simulink model "HallSensorTest"  (R2023b)
settings: Solver=FixedStepAuto  StartTime=0.0  StopTime=inf  FixedStep=0.01  RelTol=1e-3  EnableMultiTasking=on
libraries: aerolibconvert2 x1, simulink x1
settings Model: SimulationMode=external  ExtModeTrigDuration=2  Creator=sword  LastModifiedBy=sword
settings SolverCC: AutoInsertRateTranBlk=on
settings DataIOCC: SaveFormat=StructureWithTime  DSMLogging=off
settings OptimizationCC: DefaultUnderspecifiedDataType=single  EnhancedBackFolding=on  PassReuseOutputArgsAs=Individual arguments  ZeroExternalMemoryAtStartup=off  ZeroInternalMemoryAtStartup=off  MaxStackSize=64  OptimizeBlockOrder=speed  DifferentSizesBufferReuse=on  OptimizationCustomize=off  EfficientTunableParamExpr=on
settings DebuggingCC: MultiTaskDSMMsg=none  ParameterPrecisionLossMsg=none  ParameterTunabilityLossMsg=error
settings HardwareCC: ProdBitPerInt=16  ProdBitPerPointer=16  ProdBitPerSizeT=16  ProdBitPerPtrDiffT=16  ProdLargestAtomicFloat=None  ProdWordSize=8  ProdHWDeviceType=Atmel->AVR
settings SFSimCC: MATLABDynamicMemAlloc=off
settings RTWCC: Description=Embedded Coder  SystemTargetFile=ert.tlc  HardwareBoard=Arduino Mega ADK  TemplateMakefile=ert_default_tmf  Toolchain=Arduino AVR  BuildConfiguration=Faster Runs
settings CodeAppCC: ForceParamTrailComments=on  IgnoreCustomStorageClasses=off  OperatorAnnotations=on  SimulinkDataObjDesc=on  SFDataObjDesc=on  InsertBlockDesc=on
settings ERTTargetCC: SupportContinuousTime=on  SupportNonInlinedSFcns=on  SupportVariableSizeSignals=on  ExtMode=on  ExtModeTransport=3  ExtModeStaticAlloc=on  ExtModeAutomaticAllocSize=off  ExtModeStaticAllocSize=2048  ExtModeMexFile=ext_xcp  ExtModeMexArgs=0 6 115200  ExtModeIntrfLevel=Level2 - Open

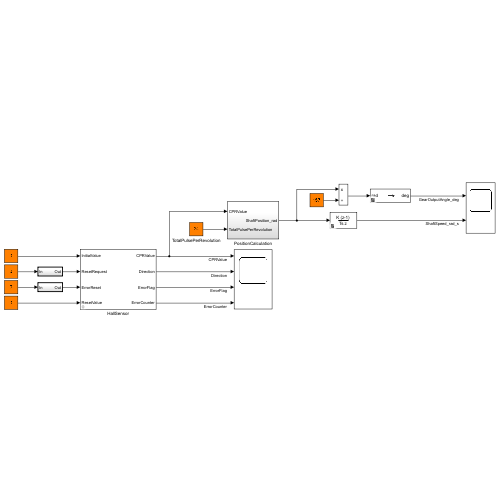
[thumbnail: Simulink's stored preview of the top-level diagram]
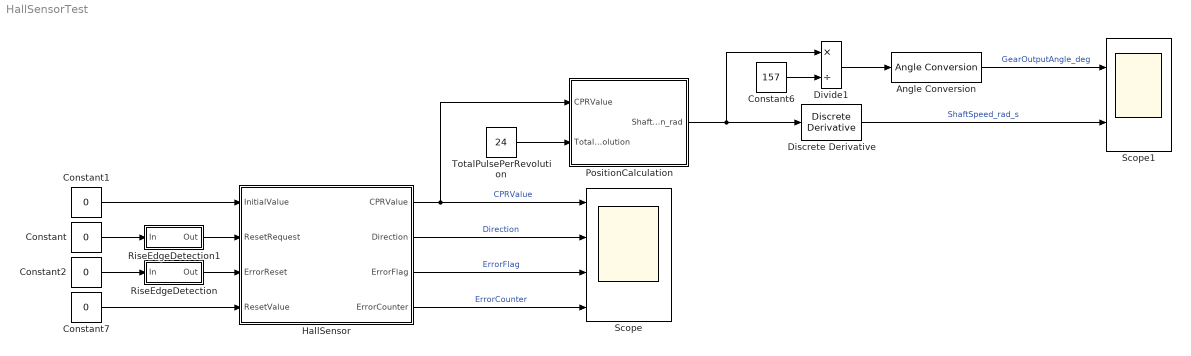
== system HallSensorTest ==
  Angle Conversion : aerolibconvert2/Angle Conversion  IU=rad  OU=deg
  Constant : Constant  Value=0  OutDataTypeStr=boolean  SampleTime=-1
  Constant1 : Constant  Value=0  OutDataTypeStr=int32  SampleTime=-1
  Constant2 : Constant  Value=0  OutDataTypeStr=boolean  SampleTime=-1
  Constant6 : Constant  Value=157  OutDataTypeStr=Inherit: Inherit via back propagation  SampleTime=-1
  Constant7 : Constant  Value=0  OutDataTypeStr=int32  SampleTime=-1
  Discrete Derivative : simulink/Discrete/Discrete Derivative  gainval=1.0  ICPrevScaledInput=0.0  OutMin=[]  OutMax=[]  OutDataType=fixdt(1, 16)  OutScaling=2^-10  RndMeth=Zero  DoSatur=on
  Divide1 : Product  Inputs=*/
  HallSensor : Subsystem  mask(HallSensorBlock){HallAPinNum=2, HallBPinNum=3, HallCPinNum=21}
      mask prompts: HallAPinNum "Pin Number of Hall A Input:"; HallBPinNum "Pin Number of Hall B Input:"; HallCPinNum "Pin Number of Hall C Input:"
      mask help:
      | This device driver block enables you to interface Hall Sensors in BLDCM and provides you CPR value, direction and other diagnostics related information.
      | This block is prepared for Arduino Mega Board.
      |
      | Information about I/Os,
      |
      | Inputs:
      | (1)Initial CPR value(int32)
      | (2)Hall sesnor reset request(boolean)
      | (3)CPR value after reset(int32)
      | (4)Transition error reset request(boolean)
      |
      | Outputs:
      | (1)Calculated CPR value(int32)
      | (2)Direction of rotation(int8)
      | (3)Transition error flag(boolean)
      | (4)Transition error counter(uint32)
      |
      | The Hall Sensor outputs must be connected to any 3 interrupt pins of the Arduino MEGA Board.
      | The interrupt pins are: 2, 3, 21, 20, 19 and 18.
      mask Help:
      | Check Simulink support package documentation for more information.
      | Also, check Arduino Mega Board documentations.
      | 
      | Author: Mehmet Kılıç
      | Github: https://github.com/saibermehmet
      | LinkedIn: https://www.linkedin.com/in/swmt
  PositionCalculation : Subsystem
  RiseEdgeDetection : Subsystem  TreatAsAtomicUnit=on
      settings: RTWSystemCode=Inline
  RiseEdgeDetection1 : Subsystem  TreatAsAtomicUnit=on
      settings: RTWSystemCode=Inline
  Scope : Scope  NumInputPorts=4
  Scope1 : Scope  NumInputPorts=2
  TotalPulsePerRevolution : Constant  Value=24  OutDataTypeStr=Inherit: Inherit via back propagation  SampleTime=-1
  wires:
  Constant6/1 -> Divide1/2
  Divide1/1 -> Angle Conversion/1
  Angle Conversion/1 -> Scope1/1  "GearOutputAngle_deg"
  Discrete Derivative/1 -> Scope1/2  "ShaftSpeed_rad_s"
  HallSensor/1(CPRValue) -> Scope/1, PositionCalculation/1(CPRValue)  "CPRValue"
  Constant/1 -> RiseEdgeDetection1/1(In)
  Constant1/1 -> HallSensor/1(InitialValue)
  Constant2/1 -> RiseEdgeDetection/1(In)
  Constant7/1 -> HallSensor/4(ResetValue)
  HallSensor/3(ErrorFlag) -> Scope/3  "ErrorFlag"
  HallSensor/4(ErrorCounter) -> Scope/4  "ErrorCounter"
  HallSensor/2(Direction) -> Scope/2  "Direction"
  RiseEdgeDetection/1(Out) -> HallSensor/3(ErrorReset)
  RiseEdgeDetection1/1(Out) -> HallSensor/2(ResetRequest)
  PositionCalculation/1(ShaftPosition_rad) -> Discrete Derivative/1, Divide1/1
  TotalPulsePerRevolution/1 -> PositionCalculation/2(TotalPulsePerRevolution)

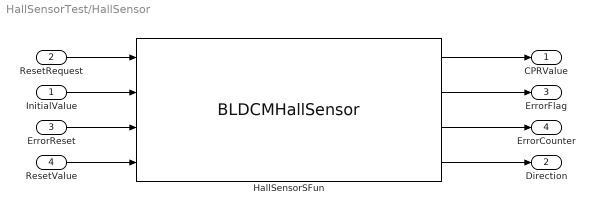
== system HallSensorTest/HallSensor ==
  InitialValue : Inport
  ResetRequest : Inport  Port=2
  ErrorReset : Inport  Port=3
  ResetValue : Inport  Port=4
  HallSensorSFun : S-Function  FunctionName=BLDCMHallSensor  Parameters=HallAPinNum,HallBPinNum,HallCPinNum  SFunctionModules=BLDCMHallSensor_wrapper.c  SFunctionDeploymentMode=off  EnableBusSupport=off  mask(S-Function Builder){}
      mask help: Simulink:masks:SFunctionBuilder_MD
      mask init:
      | val = [[.9  0.75 0.75 1 1 .9 .9 1]',[1 1 0.75 0.75 .9 .9 1 .9]'];try , sys = get_param(gcb,'SfunBuilderFcnName');if isempty(sys), sys = get_param(gcb,'FunctionName'); end,catch, sys = get_param(gcb,'FunctionName'); end
      settings: CopyFcn=set_param(gcbh,'LinkStatus','none')  OpenFcn=sfunctionwizard(gcbh)
      mask Display:
      | plot(val(:,1),val(:,2))
      | disp(sys)
      | port_label('input',1,'CPRValueResetRequest_b8')
      | port_label('input',2,'InitialCPRValue_s32')
      | port_label('input',3,'TransitionErrorReset_b8')
      | port_label('input',4,'CPRResetValue_s32')
      | port_label('output',1,'TransitionCPRValue_s32')
      | port_label('output',2,'TransitionErrorFlag_b8')
      | port_label('output',3,'TransitionErrorCounter_u32')
      | port_label('output',4,'BLDCMDirection_s8')
  CPRValue : Outport
  Direction : Outport  Port=2
  ErrorFlag : Outport  Port=3
  ErrorCounter : Outport  Port=4
  wires:
  HallSensorSFun/2 -> ErrorFlag/1
  InitialValue/1 -> HallSensorSFun/2
  ResetValue/1 -> HallSensorSFun/4
  HallSensorSFun/1 -> CPRValue/1
  HallSensorSFun/4 -> Direction/1
  ResetRequest/1 -> HallSensorSFun/1
  ErrorReset/1 -> HallSensorSFun/3
  HallSensorSFun/3 -> ErrorCounter/1

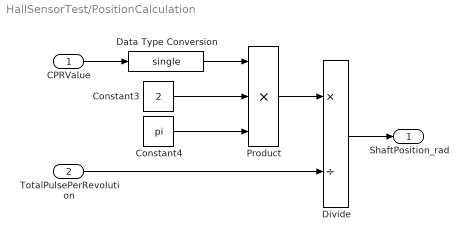
== system HallSensorTest/PositionCalculation ==
  CPRValue : Inport
  TotalPulsePerRevolution : Inport  Port=2
  Constant3 : Constant  Value=2  OutDataTypeStr=Inherit: Inherit via back propagation  SampleTime=-1
  Constant4 : Constant  Value=pi  OutDataTypeStr=Inherit: Inherit via back propagation  SampleTime=-1
  Data Type Conversion : DataTypeConversion  OutDataTypeStr=single
  Divide : Product  Inputs=*/
  Product : Product  Inputs=3  InputSameDT=on  RndMeth=Zero  SaturateOnIntegerOverflow=on
  ShaftPosition_rad : Outport
  wires:
  Product/1 -> Divide/1
  Data Type Conversion/1 -> Product/1
  Constant3/1 -> Product/2
  Constant4/1 -> Product/3
  CPRValue/1 -> Data Type Conversion/1
  Divide/1 -> ShaftPosition_rad/1
  TotalPulsePerRevolution/1 -> Divide/2

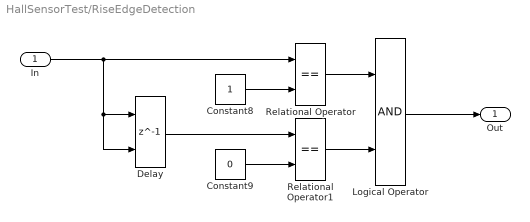
== system HallSensorTest/RiseEdgeDetection ==
  In : Inport
  Constant8 : Constant  OutDataTypeStr=boolean  SampleTime=-1
  Constant9 : Constant  Value=0  OutDataTypeStr=boolean  SampleTime=-1
  Delay : Delay  DelayLength=1  InitialConditionSource=Input port
      settings: InputPortMap=u0,p4
  Logical Operator : Logic  OutDataTypeStr=boolean
  Relational Operator : RelationalOperator  Operator===  OutDataTypeStr=boolean  RndMeth=Zero
  Relational Operator1 : RelationalOperator  Operator===  OutDataTypeStr=boolean  RndMeth=Zero
  Out : Outport
  wires:
  Constant8/1 -> Relational Operator/2
  Constant9/1 -> Relational Operator1/2
  Relational Operator/1 -> Logical Operator/1
  Relational Operator1/1 -> Logical Operator/2
  In/1 -> Delay/2, Delay/1, Relational Operator/1
  Delay/1 -> Relational Operator1/1
  Logical Operator/1 -> Out/1

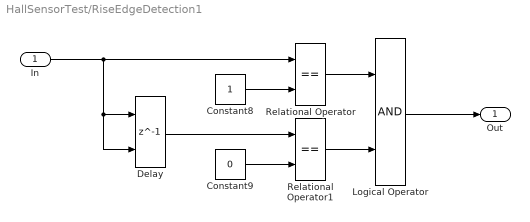
== system HallSensorTest/RiseEdgeDetection1 ==
  In : Inport
  Constant8 : Constant  OutDataTypeStr=boolean  SampleTime=-1
  Constant9 : Constant  Value=0  OutDataTypeStr=boolean  SampleTime=-1
  Delay : Delay  DelayLength=1  InitialConditionSource=Input port
      settings: InputPortMap=u0,p4
  Logical Operator : Logic  OutDataTypeStr=boolean
  Relational Operator : RelationalOperator  Operator===  OutDataTypeStr=boolean  RndMeth=Zero
  Relational Operator1 : RelationalOperator  Operator===  OutDataTypeStr=boolean  RndMeth=Zero
  Out : Outport
  wires:
  Logical Operator/1 -> Out/1
  Delay/1 -> Relational Operator1/1
  In/1 -> Relational Operator/1, Delay/1, Delay/2
  Relational Operator1/1 -> Logical Operator/2
  Relational Operator/1 -> Logical Operator/1
  Constant9/1 -> Relational Operator1/2
  Constant8/1 -> Relational Operator/2
